simulink library "VehDynaPlayGround"  (R2024b)
settings: Solver=VariableStepAuto  StartTime=0.0  StopTime=10.0  RelTol=1e-3
undefined symbols (not defined in the file or in its folder): A_F, C_af, C_ar, C_d, f, g, h_aero, h_gc, InitialX, InitialY, Iz, lf, lr, m, Nf, Nr, phi, r_stat, r_w, rho, theta, V_wind
libraries: slpidlib x5
(part 1 of 3)
settings Model: Creator=headl  LastModifiedBy=headl

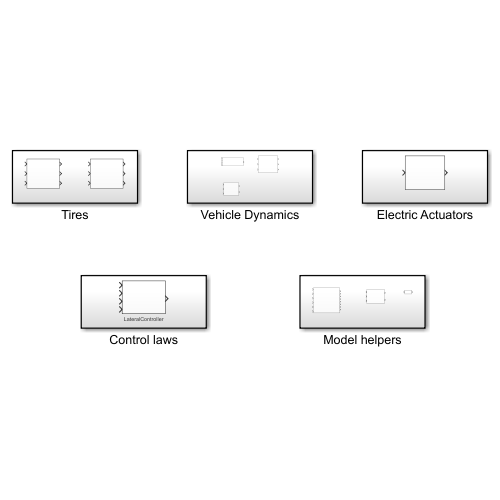
[thumbnail: Simulink's stored preview of the top-level diagram]
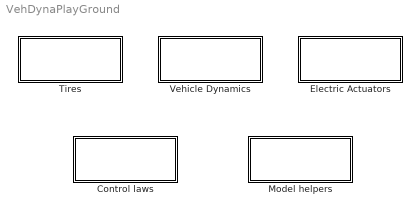
== system VehDynaPlayGround ==
  Control laws : Subsystem
  Electric Actuators : Subsystem
  Model helpers : Subsystem
  Tires : Subsystem
  Vehicle Dynamics : Subsystem

== system VehDynaPlayGround/Control laws ==
  LateralController : Subsystem  Variant=on  VariantControlMode=label  LabelModeActiveChoice=PID controller
      mask Display: image('$imagefile'); % Use "Edit Image" on toolstrip to change.

== system VehDynaPlayGround/Electric Actuators ==
  SteeringActuator : Subsystem  Variant=on  VariantControlMode=label  LabelModeActiveChoice=BLDC electric motor

== system VehDynaPlayGround/Model helpers ==
  CoordConvertRotation : Subsystem
      mask Display: image('$imagefile'); % Use "Edit Image" on toolstrip to change.
  GetRefference : MATLAB Function  TreatAsAtomicUnit=on  SystemSampleTime=0.05
  Wrap2pi : MATLAB Function  TreatAsAtomicUnit=on

== system VehDynaPlayGround/Tires ==
  Tyre ModelV1 : Subsystem
      mask Display: image('tire1_1.png');
  Tyre ModelV2 : Subsystem
      mask Display: image('$imagefile'); % Use "Edit Image" on toolstrip to change.

== system VehDynaPlayGround/Vehicle Dynamics ==
  LateralDynamics : Subsystem  Variant=on  VariantControlMode=label  LabelModeActiveChoice=Simplified Model
  LongitudinalDynamics : MATLAB Function  TreatAsAtomicUnit=on
  Transmission : MATLAB Function  TreatAsAtomicUnit=on

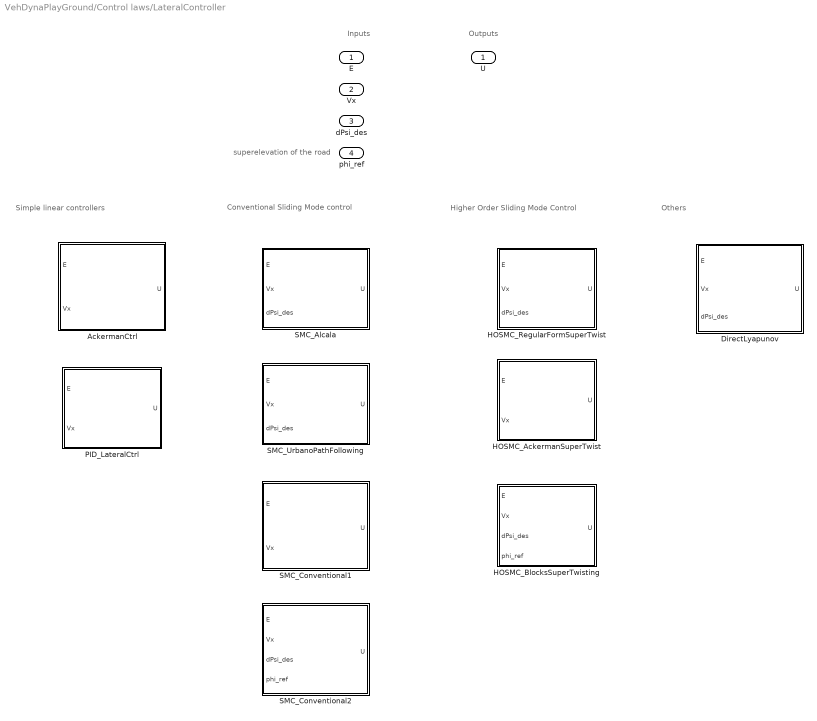
== system VehDynaPlayGround/Control laws/LateralController ==
  note: Others
  note: Higher Order Sliding Mode Control
  note: Conventional Sliding Mode control
  note: Simple linear controllers
  note: Outputs
  note: Inputs
  note: superelevation of the road
  E : Inport
  Vx : Inport  Port=2
  dPsi_des : Inport  Port=3
  phi_ref : Inport  Port=4
  AckermanCtrl : MATLAB Function  TreatAsAtomicUnit=on  VariantControl=Ackerman error feedback
  DirectLyapunov : MATLAB Function  TreatAsAtomicUnit=on  VariantControl=Direct Lyapunov Alcala et al.
  HOSMC_AckermanSuperTwist : Subsystem  VariantControl="HOSM  Ackerman + super twisting"
      mask Display: image('$imagefile'); % Use "Edit Image" on toolstrip to change.
  HOSMC_BlocksSuperTwisting : Subsystem  VariantControl=HOSM error feedback block +super twisting
      mask Display: image('$imagefile'); % Use "Edit Image" on toolstrip to change.
  HOSMC_RegularFormSuperTwist : Subsystem  VariantControl=HOSM regular form +super twisting
      mask Display: image('$imagefile'); % Use "Edit Image" on toolstrip to change.
  PID_LateralCtrl : Subsystem  VariantControl=PID controller
      mask Display: image('$imagefile'); % Use "Edit Image" on toolstrip to change.
  SMC_Alcala : Subsystem  VariantControl=Sliding mode Alcala et al.
      mask Display: image('$imagefile'); % Use "Edit Image" on toolstrip to change.
  SMC_Conventional1 : MATLAB Function  TreatAsAtomicUnit=on  VariantControl=SMC conventional V1
  SMC_Conventional2 : MATLAB Function  TreatAsAtomicUnit=on  VariantControl=SMC conventional V2
  SMC_UrbanoPathFollowing : Subsystem  VariantControl=Sliding mode Urbano path following
      mask Display: image('$imagefile'); % Use "Edit Image" on toolstrip to change.
  U : Outport

== system VehDynaPlayGround/Electric Actuators/SteeringActuator ==
  dd_ref : Inport
  BLDC_AngleCtrl : Subsystem  VariantControl=BLDC electric motor
      mask Display: image('$imagefile'); % Use "Edit Image" on toolstrip to change.
  NoActuator : Subsystem  VariantControl=No Actuator
  genericTransferFunction : Subsystem  VariantControl=Generic transfer function
      mask Display: image('$imagefile'); % Use "Edit Image" on toolstrip to change.
  dd_ctrl : Outport

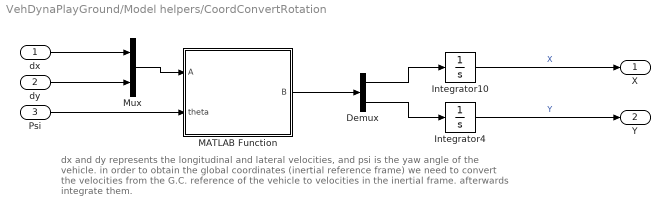
== system VehDynaPlayGround/Model helpers/CoordConvertRotation ==
  note: dx and dy represents the longitudinal and lateral velocities, and psi is the yaw angle of the vehicle. in order to obtain the global coordinates (inertial reference frame) we need to convert the velocities from the G.C. reference of the vehicle to velocities in the inertial frame. afterwards integrate them.
  dx : Inport
  dy : Inport  Port=2
  Psi : Inport  Port=3
  Demux : Demux  Outputs=2
  Integrator10 : Integrator  InitialCondition=InitialX
  Integrator4 : Integrator  InitialCondition=InitialY
  MATLAB Function : MATLAB Function  TreatAsAtomicUnit=on
  Mux : Mux  Inputs=2
  X : Outport  VectorParamsAs1DForOutWhenUnconnected=off
  Y : Outport  Port=2  VectorParamsAs1DForOutWhenUnconnected=off
  wires:
  Integrator10/1 -> X/1  "X"
  Integrator4/1 -> Y/1  "Y"
  Psi/1 -> MATLAB Function/2(theta)
  dx/1 -> Mux/1
  dy/1 -> Mux/2
  Mux/1 -> MATLAB Function/1(A)
  MATLAB Function/1(B) -> Demux/1
  Demux/1 -> Integrator10/1
  Demux/2 -> Integrator4/1

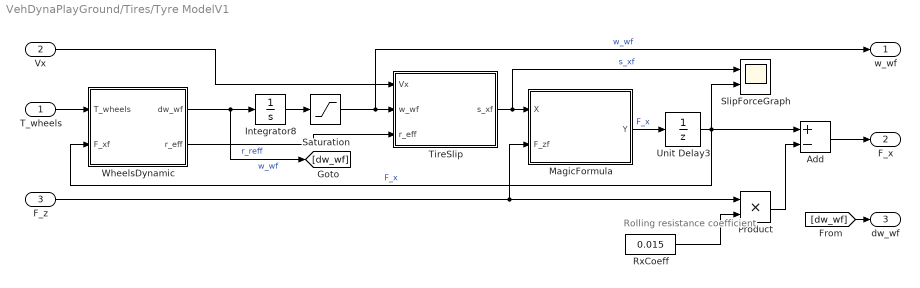
== system VehDynaPlayGround/Tires/Tyre ModelV1 ==
  note: Rolling resistance
      | coefficient
  T_wheels : Inport
  Vx : Inport  Port=2
  F_z : Inport  Port=3
  Add : Sum  Inputs=+-
  Integrator8 : Integrator
  MagicFormula : MATLAB Function  TreatAsAtomicUnit=on
  Product : Product
  RxCoeff : Constant  Value=0.015
  Saturation : Saturate  UpperLimit=100000  LowerLimit=0
  SlipForceGraph : Scope  NumInputPorts=2
  TireSlip : MATLAB Function  TreatAsAtomicUnit=on
  Unit Delay3 : UnitDelay  SampleTime=-1  HasFrameUpgradeWarning=on
  WheelsDynamic : MATLAB Function  TreatAsAtomicUnit=on
  w_wf : Outport
  F_x : Outport  Port=2
  dw_wf : Outport  Port=3
  wires:
  T_wheels/1 -> WheelsDynamic/1(T_wheels)
  Saturation/1 -> w_wf/1, TireSlip/2(w_wf)  "w_wf"
  WheelsDynamic/2(r_eff) -> TireSlip/3(r_eff)  "r_reff"
  MagicFormula/1(Y) -> Unit Delay3/1  "F_x"
  TireSlip/1(s_xf) -> SlipForceGraph/1, MagicFormula/1(X)  "s_xf"
  Integrator8/1 -> Saturation/1
  Vx/1 -> TireSlip/1(Vx)
  [dw_wf] -> dw_wf/1
  WheelsDynamic/1(dw_wf) -> [dw_wf], Integrator8/1  "w_wf"
  Add/1 -> F_x/1
  Product/1 -> Add/2
  F_z/1 -> Product/1, MagicFormula/2(F_zf)
  Unit Delay3/1 -> Add/1, SlipForceGraph/2, WheelsDynamic/2(F_xf)  "F_x"
  RxCoeff/1 -> Product/2

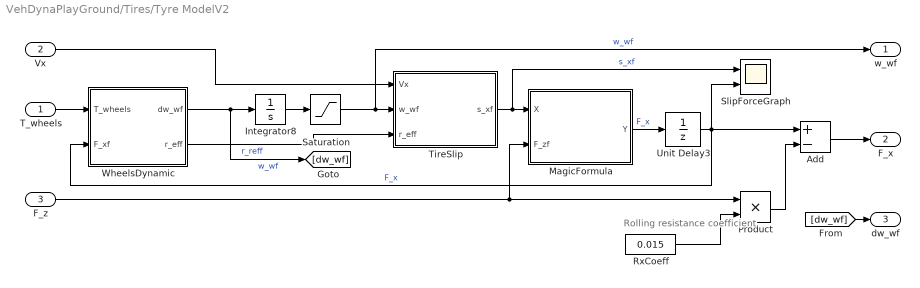
== system VehDynaPlayGround/Tires/Tyre ModelV2 ==
  note: Rolling resistance
      | coefficient
  T_wheels : Inport
  Vx : Inport  Port=2
  F_z : Inport  Port=3
  Add : Sum  Inputs=+-
  Integrator8 : Integrator
  MagicFormula : MATLAB Function  TreatAsAtomicUnit=on
  Product : Product
  RxCoeff : Constant  Value=0.015
  Saturation : Saturate  UpperLimit=100000  LowerLimit=0
  SlipForceGraph : Scope  NumInputPorts=2
  TireSlip : MATLAB Function  TreatAsAtomicUnit=on
  Unit Delay3 : UnitDelay  SampleTime=-1  HasFrameUpgradeWarning=on
  WheelsDynamic : MATLAB Function  TreatAsAtomicUnit=on
  w_wf : Outport
  F_x : Outport  Port=2
  dw_wf : Outport  Port=3
  wires:
  T_wheels/1 -> WheelsDynamic/1(T_wheels)
  Saturation/1 -> w_wf/1, TireSlip/2(w_wf)  "w_wf"
  WheelsDynamic/2(r_eff) -> TireSlip/3(r_eff)  "r_reff"
  MagicFormula/1(Y) -> Unit Delay3/1  "F_x"
  TireSlip/1(s_xf) -> SlipForceGraph/1, MagicFormula/1(X)  "s_xf"
  Integrator8/1 -> Saturation/1
  Vx/1 -> TireSlip/1(Vx)
  [dw_wf] -> dw_wf/1
  WheelsDynamic/1(dw_wf) -> [dw_wf], Integrator8/1  "w_wf"
  Add/1 -> F_x/1
  Product/1 -> Add/2
  F_z/1 -> Product/1, MagicFormula/2(F_zf)
  Unit Delay3/1 -> Add/1, SlipForceGraph/2, WheelsDynamic/2(F_xf)  "F_x"
  RxCoeff/1 -> Product/2

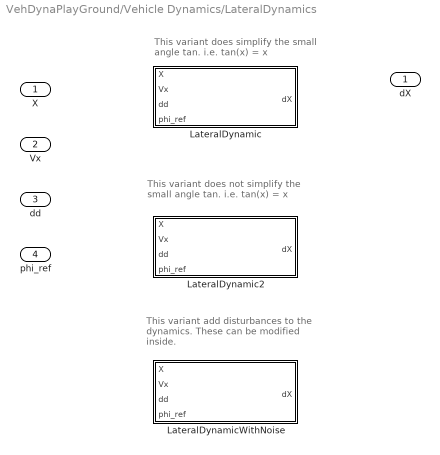
== system VehDynaPlayGround/Vehicle Dynamics/LateralDynamics ==
  note: This variant does not simplify the small angle tan. i.e. tan(x) = x
  note: This variant does simplify the small angle tan. i.e. tan(x) = x
  note: This variant add disturbances to the dynamics. These can be modified inside.
  X : Inport
  Vx : Inport  Port=2
  dd : Inport  Port=3
  phi_ref : Inport  Port=4
  LateralDynamic : MATLAB Function  TreatAsAtomicUnit=on  VariantControl=Simplified Model
  LateralDynamic2 : MATLAB Function  TreatAsAtomicUnit=on  VariantControl=Not Simplified Model
  LateralDynamicWithNoise : Subsystem  VariantControl=Lateral dynamic with disturbances
      mask Display: image('$imagefile'); % Use "Edit Image" on toolstrip to change.
  dX : Outport

== system VehDynaPlayGround/Control laws/LateralController/HOSMC_AckermanSuperTwist ==
  E : Inport
  Vx : Inport  Port=2
  HOSMC_AckermanSuperTwis1 : MATLAB Function  TreatAsAtomicUnit=on  VariantControl=SMC conventional
  Integrator1 : Integrator
  U : Outport
  wires:
  HOSMC_AckermanSuperTwis1/1(U) -> U/1
  E/1 -> HOSMC_AckermanSuperTwis1/1(E)
  Vx/1 -> HOSMC_AckermanSuperTwis1/2(Vx)
  HOSMC_AckermanSuperTwis1/2(dMu1) -> Integrator1/1
  Integrator1/1 -> HOSMC_AckermanSuperTwis1/3(Mu1)

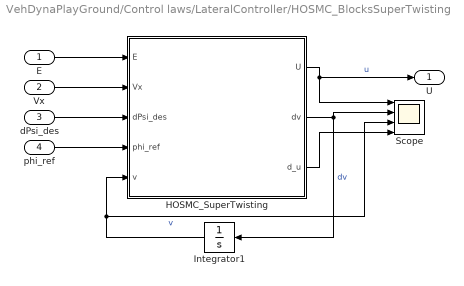
== system VehDynaPlayGround/Control laws/LateralController/HOSMC_BlocksSuperTwisting ==
  E : Inport
  Vx : Inport  Port=2
  dPsi_des : Inport  Port=3
  phi_ref : Inport  Port=4
  HOSMC_SuperTwisting : MATLAB Function  TreatAsAtomicUnit=on  VariantControl=SMC conventional
  Integrator1 : Integrator
  Scope : Scope  NumInputPorts=4
  U : Outport
  wires:
  HOSMC_SuperTwisting/1(U) -> U/1, Scope/1  "u"
  E/1 -> HOSMC_SuperTwisting/1(E)
  Vx/1 -> HOSMC_SuperTwisting/2(Vx)
  HOSMC_SuperTwisting/2(dv) -> Integrator1/1, Scope/2  "dv"
  Integrator1/1 -> Scope/3, HOSMC_SuperTwisting/5(v)  "v"
  dPsi_des/1 -> HOSMC_SuperTwisting/3(dPsi_des)
  phi_ref/1 -> HOSMC_SuperTwisting/4(phi_ref)
  HOSMC_SuperTwisting/3(d_u) -> Scope/4

== system VehDynaPlayGround/Control laws/LateralController/HOSMC_RegularFormSuperTwist ==
  E : Inport
  Vx : Inport  Port=2
  dPsi_des : Inport  Port=3
  HOSMC_RegularFormSuperTwist : MATLAB Function  TreatAsAtomicUnit=on  VariantControl=SMC conventional
  Integrator1 : Integrator
  Scope : Scope  NumInputPorts=3
  U : Outport
  wires:
  HOSMC_RegularFormSuperTwist/1(U) -> Scope/1, U/1
  E/1 -> HOSMC_RegularFormSuperTwist/1(E)
  Vx/1 -> HOSMC_RegularFormSuperTwist/2(Vx)
  HOSMC_RegularFormSuperTwist/2(dMu1) -> Integrator1/1, Scope/2
  Integrator1/1 -> Scope/3, HOSMC_RegularFormSuperTwist/4(Mu1)
  dPsi_des/1 -> HOSMC_RegularFormSuperTwist/3(dPsi_des)

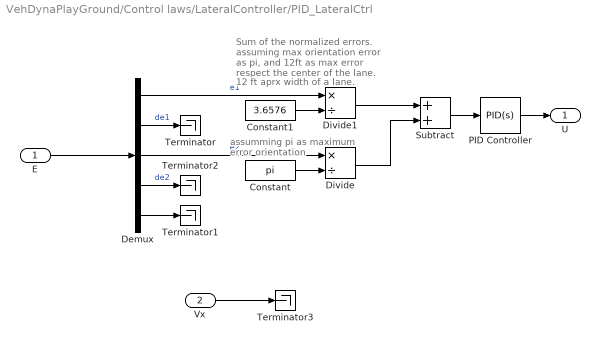
== system VehDynaPlayGround/Control laws/LateralController/PID_LateralCtrl ==
  note: Sum of the normalized errors. assuming max orientation error as pi, and 12ft as max error respect the center of the lane.
  note: assumming pi as maximum error orientation
  note: 12 ft aprx width of a lane.
  E : Inport
  Vx : Inport  Port=2
  Constant : Constant  Value=pi
  Constant1 : Constant  Value=3.6576
  Demux : Demux  Outputs=5
  Divide : Product  Inputs=*/
  Divide1 : Product  Inputs=*/
  PID Controller : slpidlib/PID Controller  Controller=PID  Form=Parallel  TimeDomain=Continuous-time  UseExternalTs=off  SampleTime=-1  IntegratorMethod=Forward Euler  FilterMethod=Forward Euler  ControllerParametersSource=internal  P=-10.4366715621745  I=-1.38825323496777  UseKiTs=off  D=1.48027109324461  UseExternalDerivativeSource=off  N=1.62687524156854  UseFilter=on  TunerSelectOption=Transfer Function Based (PID Tuner App)  InitialConditionSource=internal  InitialConditionForIntegrator=0  InitialConditionForFilter=0  DifferentiatorICPrevScaledInput=0  ExternalReset=none  TrackingMode=off  Kt=1  LimitOutput=off  SatLimitsSource=internal  UpperSaturationLimit=inf  LowerSaturationLimit=-inf  LinearizeAsGain=on  AntiWindupMode=none  Kb=1  LimitIntegrator=off  UpperIntegratorSaturationLimit=inf  LowerIntegratorSaturationLimit=-inf  POutMin=[]  POutMax=[]  IOutMin=[]  IOutMax=[]  DOutMin=[]  DOutMax=[]  NOutMin=[]  NOutMax=[]  SumOutMin=[]  SumOutMax=[]  SaturationOutMin=[]  SaturationOutMax=[]  PParamMin=[]  PParamMax=[]  IParamMin=[]  IParamMax=[]  DParamMin=[]  DParamMax=[]  NParamMin=[]  NParamMax=[]  KbParamMin=[]  KbParamMax=[]  KtParamMin=[]  KtParamMax=[]  KbOutMin=[]  KbOutMax=[]  KtOutMin=[]  KtOutMax=[]  IntegratorOutMin=[]  IntegratorOutMax=[]  FilterOutMin=[]  FilterOutMax=[]  SumI1OutMin=[]  SumI1OutMax=[]  SumI2OutMin=[]  SumI2OutMax=[]  SumI3OutMin=[]  SumI3OutMax=[]  SumI4OutMin=[]  SumI4OutMax=[]  SumDOutMin=[]  SumDOutMax=[]  DifferentiatorOutMin=[]  DifferentiatorOutMax=[]  FilterDiffOutCoefMin=[]  FilterDiffOutCoefMax=[]  ReciprocalOutMin=[]  ReciprocalOutMax=[]  SumDenOutMin=[]  SumDenOutMax=[]  SumNumOutMin=[]  SumNumOutMax=[]  DivideOutMin=[]  DivideOutMax=[]  UdiffTsProdOutMin=[]  UdiffTsProdOutMax=[]  NTsProdOutMin=[]  NTsProdOutMax=[]  UintegralTsProdOutMin=[]  UintegralTsProdOutMax=[]  UngainTsProdOutMin=[]  UngainTsProdOutMax=[]  ClampingZeroOutDataTypeStr=Inherit: Inherit via back propagation  ClampingZeroOutMin=[]  ClampingZeroOutMax=[]  FilterDenConstantOutDataTypeStr=Inherit: Inherit via back propagation  FilterDenConstantOutMin=[]  FilterDenConstantOutMax=[]  PCopyOutDataTypeStr=Inherit: Inherit via back propagation  PCopyOutMin=[]  PCopyOutMax=[]  NCopyOutDataTypeStr=Inherit: Inherit via back propagation  NCopyOutMin=[]  NCopyOutMax=[]  IntegratorContinuousStateAttributes=''  IntegratorStateMustResolveToSignalObject=off  IntegratorRTWStateStorageClass=Auto  FilterContinuousStateAttributes=''  FilterStateMustResolveToSignalObject=off  FilterRTWStateStorageClass=Auto  ParallelPVariant=InternalParameters  IdealPVariant=Disabled  IVariant=InternalParameters  DVariant=InternalParameters  IntegratorVariant=Continuous  SatVariant=Disabled  AWVariant=Passthrough  PCopyVariant=Disabled  TRVariant=Disabled  FdbkBlocksVariant=Forward  IdealPFdbkVariant=Disabled  SatFdbkVariant=Disabled  DerivativeFilterVariant=ContFilter  NVariant=InternalParameters  NCopyVariant=Disabled  FilterICVariant=InternalICsFilter  IntegratorICVariant=InternalICs  ExternalResetVariant=Disabled  TRSumVariant=Passthrough  SumFdbkVariant=Disabled  SumVariant=Sum_PID  TsampFilterVariant=InternalTs  TsampNgainVariant=Passthrough  TsampIntegralVariant=Disabled_SignalSpec  ExternalSaturationOutDataTypeStr=Inherit: Same as second input  DerivativeSourceVariant=ErrorSignal  PreIntVariant=InternalPreInt
  Subtract : Sum
  Terminator{,1..3} (4 alike) : Terminator
  U : Outport
  wires:
  E/1 -> Demux/1
  Demux/2 -> Terminator/1  "de1"
  Demux/4 -> Terminator2/1  "de2"
  Vx/1 -> Terminator3/1
  Subtract/1 -> PID Controller/1
  PID Controller/1 -> U/1
  Demux/3 -> Divide/1  "e2"
  Divide/1 -> Subtract/2
  Constant/1 -> Divide/2
  Demux/1 -> Divide1/1  "e1"
  Constant1/1 -> Divide1/2
  Divide1/1 -> Subtract/1
  Demux/5 -> Terminator1/1

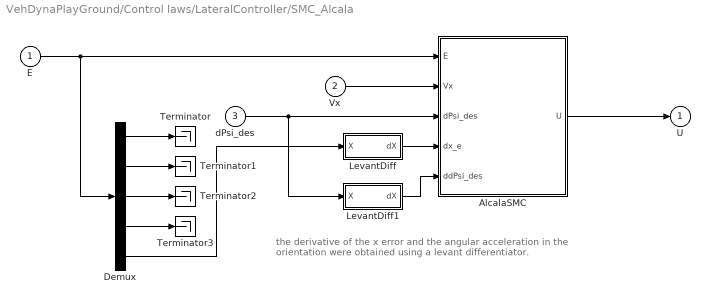
== system VehDynaPlayGround/Control laws/LateralController/SMC_Alcala ==
  note: the derivative of the x error and the angular acceleration in the orientation were obtained using a levant differentiator.
  E : Inport
  Vx : Inport  Port=2
  dPsi_des : Inport  Port=3
  AlcalaSMC : MATLAB Function  TreatAsAtomicUnit=on  VariantControl=Sliding mode Ctrl 1
  Demux : Demux  Outputs=5
  LevantDiff : Subsystem  mask{lambda1=60, alpha1=2000}
      mask prompts: lambda1 "Lambda :"; alpha1 "Alpha    :"
      mask help: Levant differenciator
      mask Help: This is based on Levant A. (1998). Robust exact differentiation via sliding mode technique. Automatica, 34(3), 379-384
  LevantDiff1 : Subsystem  mask{lambda1=60, alpha1=2000}
      mask prompts: lambda1 "Lambda :"; alpha1 "Alpha    :"
      mask help: Levant differenciator
      mask Help: This is based on Levant A. (1998). Robust exact differentiation via sliding mode technique. Automatica, 34(3), 379-384
  Terminator{,1..3} (4 alike) : Terminator
  U : Outport
  wires:
  E/1 -> Demux/1, AlcalaSMC/1(E)
  Vx/1 -> AlcalaSMC/2(Vx)
  dPsi_des/1 -> LevantDiff1/1(X), AlcalaSMC/3(dPsi_des)
  AlcalaSMC/1(U) -> U/1
  Demux/1 -> Terminator/1
  Demux/2 -> Terminator1/1
  Demux/3 -> Terminator2/1
  Demux/4 -> Terminator3/1
  LevantDiff/1(dX) -> AlcalaSMC/4(dx_e)
  Demux/5 -> LevantDiff/1(X)
  LevantDiff1/1(dX) -> AlcalaSMC/5(ddPsi_des)

== system VehDynaPlayGround/Control laws/LateralController/SMC_UrbanoPathFollowing ==
  E : Inport
  Vx : Inport  Port=2
  dPsi_des : Inport  Port=3
  Integrator : Integrator
  SMC_UrbanoPathFollowing : MATLAB Function  TreatAsAtomicUnit=on  VariantControl=Sliding mode Urbano Path Following
  U : Outport
  wires:
  SMC_UrbanoPathFollowing/1(U) -> U/1
  E/1 -> SMC_UrbanoPathFollowing/1(E)
  Vx/1 -> SMC_UrbanoPathFollowing/2(Vx)
  dPsi_des/1 -> SMC_UrbanoPathFollowing/3(dPsi_des)
  SMC_UrbanoPathFollowing/2(dd_d) -> Integrator/1
  Integrator/1 -> SMC_UrbanoPathFollowing/4(d_d)

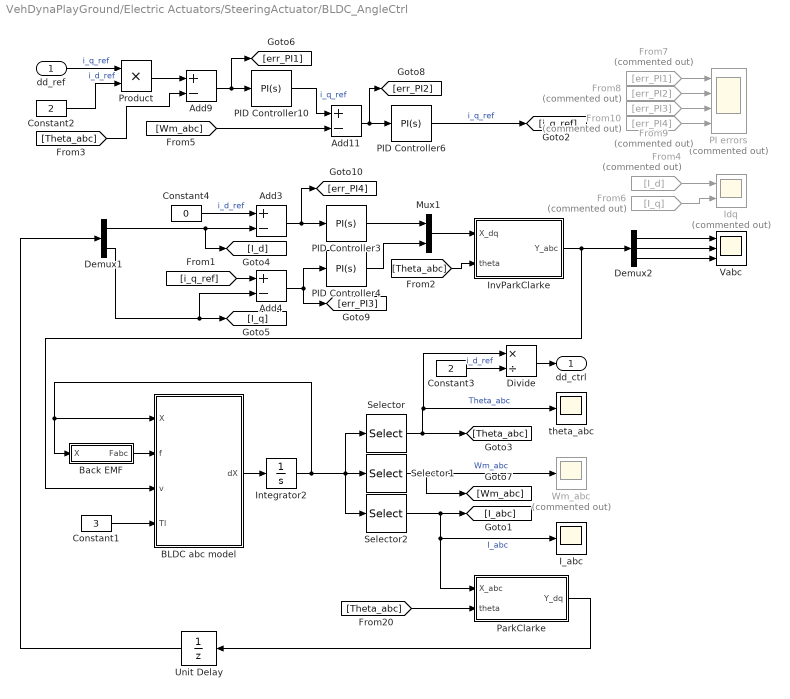
== system VehDynaPlayGround/Electric Actuators/SteeringActuator/BLDC_AngleCtrl ==
  dd_ref : Inport
  Add{3..4,9,11} (4 alike) : Sum  Inputs=+-
  BLDC abc model : MATLAB Function  TreatAsAtomicUnit=on
  Back EMF : MATLAB Function  TreatAsAtomicUnit=on
  Constant1 : Constant  Value=3
  Constant2 : Constant  Value=2
  Constant3 : Constant  Value=2
  Constant4 : Constant  Value=0
  Demux1 : Demux  Outputs=2
  Demux2 : Demux  Outputs=3
  Divide : Product  Inputs=*/
  From10 : From  Commented=on  GotoTag=err_PI4
  From4 : From  Commented=on  GotoTag=I_d
  From6 : From  Commented=on  GotoTag=I_q
  From7 : From  Commented=on  GotoTag=err_PI1
  From8 : From  Commented=on  GotoTag=err_PI2
  From9 : From  Commented=on  GotoTag=err_PI3
  I_abc : Scope
  Idq : Scope  Commented=on  NumInputPorts=2
  Integrator2 : Integrator  InitialCondition=[0;0;0;0.1;0]
  InvParkClarke : MATLAB Function  TreatAsAtomicUnit=on
  Mux1 : Mux  Inputs=2
  PI errors : Scope  Commented=on  NumInputPorts=4
  PID Controller10 : slpidlib/PID Controller  Controller=PI  Form=Parallel  TimeDomain=Continuous-time  UseExternalTs=off  SampleTime=-1  IntegratorMethod=Forward Euler  FilterMethod=Forward Euler  ControllerParametersSource=internal  P=21.2472922845302  I=1497.59558537531  UseKiTs=off  D=0  UseExternalDerivativeSource=off  N=100  UseFilter=on  TunerSelectOption=Transfer Function Based (PID Tuner App)  InitialConditionSource=internal  InitialConditionForIntegrator=0  InitialConditionForFilter=0  DifferentiatorICPrevScaledInput=0  ExternalReset=none  TrackingMode=off  Kt=1  LimitOutput=off  SatLimitsSource=internal  UpperSaturationLimit=inf  LowerSaturationLimit=-inf  LinearizeAsGain=on  AntiWindupMode=none  Kb=1  LimitIntegrator=off  UpperIntegratorSaturationLimit=inf  LowerIntegratorSaturationLimit=-inf  POutMin=[]  POutMax=[]  IOutMin=[]  IOutMax=[]  DOutMin=[]  DOutMax=[]  NOutMin=[]  NOutMax=[]  SumOutMin=[]  SumOutMax=[]  SaturationOutMin=[]  SaturationOutMax=[]  PParamMin=[]  PParamMax=[]  IParamMin=[]  IParamMax=[]  DParamMin=[]  DParamMax=[]  NParamMin=[]  NParamMax=[]  KbParamMin=[]  KbParamMax=[]  KtParamMin=[]  KtParamMax=[]  KbOutMin=[]  KbOutMax=[]  KtOutMin=[]  KtOutMax=[]  IntegratorOutMin=[]  IntegratorOutMax=[]  FilterOutMin=[]  FilterOutMax=[]  SumI1OutMin=[]  SumI1OutMax=[]  SumI2OutMin=[]  SumI2OutMax=[]  SumI3OutMin=[]  SumI3OutMax=[]  SumI4OutMin=[]  SumI4OutMax=[]  SumDOutMin=[]  SumDOutMax=[]  DifferentiatorOutMin=[]  DifferentiatorOutMax=[]  FilterDiffOutCoefMin=[]  FilterDiffOutCoefMax=[]  ReciprocalOutMin=[]  ReciprocalOutMax=[]  SumDenOutMin=[]  SumDenOutMax=[]  SumNumOutMin=[]  SumNumOutMax=[]  DivideOutMin=[]  DivideOutMax=[]  UdiffTsProdOutMin=[]  UdiffTsProdOutMax=[]  NTsProdOutMin=[]  NTsProdOutMax=[]  UintegralTsProdOutMin=[]  UintegralTsProdOutMax=[]  UngainTsProdOutMin=[]  UngainTsProdOutMax=[]  ClampingZeroOutDataTypeStr=Inherit: Inherit via back propagation  ClampingZeroOutMin=[]  ClampingZeroOutMax=[]  FilterDenConstantOutDataTypeStr=Inherit: Inherit via back propagation  FilterDenConstantOutMin=[]  FilterDenConstantOutMax=[]  PCopyOutDataTypeStr=Inherit: Inherit via back propagation  PCopyOutMin=[]  PCopyOutMax=[]  NCopyOutDataTypeStr=Inherit: Inherit via back propagation  NCopyOutMin=[]  NCopyOutMax=[]  IntegratorContinuousStateAttributes=''  IntegratorStateMustResolveToSignalObject=off  IntegratorRTWStateStorageClass=Auto  FilterContinuousStateAttributes=''  FilterStateMustResolveToSignalObject=off  FilterRTWStateStorageClass=Auto  ParallelPVariant=InternalParameters  IdealPVariant=Disabled  IVariant=InternalParameters  DVariant=Disabled  IntegratorVariant=Continuous  SatVariant=Disabled  AWVariant=Passthrough  PCopyVariant=Disabled  TRVariant=Disabled  FdbkBlocksVariant=Forward  IdealPFdbkVariant=Disabled  SatFdbkVariant=Disabled  DerivativeFilterVariant=Disabled  NVariant=Disabled  NCopyVariant=Disabled_SignalSpec  FilterICVariant=Disabled  IntegratorICVariant=InternalICs  ExternalResetVariant=Disabled  TRSumVariant=Passthrough  SumFdbkVariant=Disabled  SumVariant=Sum_PI  TsampFilterVariant=InternalTs  TsampNgainVariant=Passthrough  TsampIntegralVariant=Disabled_SignalSpec  ExternalSaturationOutDataTypeStr=Inherit: Same as second input  DerivativeSourceVariant=Disabled  PreIntVariant=InternalPreInt
  PID Controller3 : slpidlib/PID Controller  Controller=PI  Form=Parallel  TimeDomain=Continuous-time  UseExternalTs=off  SampleTime=-1  IntegratorMethod=Forward Euler  FilterMethod=Forward Euler  ControllerParametersSource=internal  P=70  I=0.3  UseKiTs=off  D=0  UseExternalDerivativeSource=off  N=100  UseFilter=on  TunerSelectOption=Transfer Function Based (PID Tuner App)  InitialConditionSource=internal  InitialConditionForIntegrator=0  InitialConditionForFilter=0  DifferentiatorICPrevScaledInput=0  ExternalReset=none  TrackingMode=off  Kt=1  LimitOutput=off  SatLimitsSource=internal  UpperSaturationLimit=inf  LowerSaturationLimit=-inf  LinearizeAsGain=on  AntiWindupMode=none  Kb=1  LimitIntegrator=off  UpperIntegratorSaturationLimit=inf  LowerIntegratorSaturationLimit=-inf  POutMin=[]  POutMax=[]  IOutMin=[]  IOutMax=[]  DOutMin=[]  DOutMax=[]  NOutMin=[]  NOutMax=[]  SumOutMin=[]  SumOutMax=[]  SaturationOutMin=[]  SaturationOutMax=[]  PParamMin=[]  PParamMax=[]  IParamMin=[]  IParamMax=[]  DParamMin=[]  DParamMax=[]  NParamMin=[]  NParamMax=[]  KbParamMin=[]  KbParamMax=[]  KtParamMin=[]  KtParamMax=[]  KbOutMin=[]  KbOutMax=[]  KtOutMin=[]  KtOutMax=[]  IntegratorOutMin=[]  IntegratorOutMax=[]  FilterOutMin=[]  FilterOutMax=[]  SumI1OutMin=[]  SumI1OutMax=[]  SumI2OutMin=[]  SumI2OutMax=[]  SumI3OutMin=[]  SumI3OutMax=[]  SumI4OutMin=[]  SumI4OutMax=[]  SumDOutMin=[]  SumDOutMax=[]  DifferentiatorOutMin=[]  DifferentiatorOutMax=[]  FilterDiffOutCoefMin=[]  FilterDiffOutCoefMax=[]  ReciprocalOutMin=[]  ReciprocalOutMax=[]  SumDenOutMin=[]  SumDenOutMax=[]  SumNumOutMin=[]  SumNumOutMax=[]  DivideOutMin=[]  DivideOutMax=[]  UdiffTsProdOutMin=[]  UdiffTsProdOutMax=[]  NTsProdOutMin=[]  NTsProdOutMax=[]  UintegralTsProdOutMin=[]  UintegralTsProdOutMax=[]  UngainTsProdOutMin=[]  UngainTsProdOutMax=[]  ClampingZeroOutDataTypeStr=Inherit: Inherit via back propagation  ClampingZeroOutMin=[]  ClampingZeroOutMax=[]  FilterDenConstantOutDataTypeStr=Inherit: Inherit via back propagation  FilterDenConstantOutMin=[]  FilterDenConstantOutMax=[]  PCopyOutDataTypeStr=Inherit: Inherit via back propagation  PCopyOutMin=[]  PCopyOutMax=[]  NCopyOutDataTypeStr=Inherit: Inherit via back propagation  NCopyOutMin=[]  NCopyOutMax=[]  IntegratorContinuousStateAttributes=''  IntegratorStateMustResolveToSignalObject=off  IntegratorRTWStateStorageClass=Auto  FilterContinuousStateAttributes=''  FilterStateMustResolveToSignalObject=off  FilterRTWStateStorageClass=Auto  ParallelPVariant=InternalParameters  IdealPVariant=Disabled  IVariant=InternalParameters  DVariant=Disabled  IntegratorVariant=Continuous  SatVariant=Disabled  AWVariant=Passthrough  PCopyVariant=Disabled  TRVariant=Disabled  FdbkBlocksVariant=Forward  IdealPFdbkVariant=Disabled  SatFdbkVariant=Disabled  DerivativeFilterVariant=Disabled  NVariant=Disabled  NCopyVariant=Disabled_SignalSpec  FilterICVariant=Disabled  IntegratorICVariant=InternalICs  ExternalResetVariant=Disabled  TRSumVariant=Passthrough  SumFdbkVariant=Disabled  SumVariant=Sum_PI  TsampFilterVariant=InternalTs  TsampNgainVariant=Passthrough  TsampIntegralVariant=Disabled_SignalSpec  ExternalSaturationOutDataTypeStr=Inherit: Same as second input  DerivativeSourceVariant=Disabled  PreIntVariant=InternalPreInt
  PID Controller4 : slpidlib/PID Controller  Controller=PI  Form=Parallel  TimeDomain=Continuous-time  UseExternalTs=off  SampleTime=-1  IntegratorMethod=Forward Euler  FilterMethod=Forward Euler  ControllerParametersSource=internal  P=70  I=0.3  UseKiTs=off  D=0  UseExternalDerivativeSource=off  N=100  UseFilter=on  TunerSelectOption=Transfer Function Based (PID Tuner App)  InitialConditionSource=internal  InitialConditionForIntegrator=0  InitialConditionForFilter=0  DifferentiatorICPrevScaledInput=0  ExternalReset=none  TrackingMode=off  Kt=1  LimitOutput=off  SatLimitsSource=internal  UpperSaturationLimit=inf  LowerSaturationLimit=-inf  LinearizeAsGain=on  AntiWindupMode=none  Kb=1  LimitIntegrator=off  UpperIntegratorSaturationLimit=inf  LowerIntegratorSaturationLimit=-inf  POutMin=[]  POutMax=[]  IOutMin=[]  IOutMax=[]  DOutMin=[]  DOutMax=[]  NOutMin=[]  NOutMax=[]  SumOutMin=[]  SumOutMax=[]  SaturationOutMin=[]  SaturationOutMax=[]  PParamMin=[]  PParamMax=[]  IParamMin=[]  IParamMax=[]  DParamMin=[]  DParamMax=[]  NParamMin=[]  NParamMax=[]  KbParamMin=[]  KbParamMax=[]  KtParamMin=[]  KtParamMax=[]  KbOutMin=[]  KbOutMax=[]  KtOutMin=[]  KtOutMax=[]  IntegratorOutMin=[]  IntegratorOutMax=[]  FilterOutMin=[]  FilterOutMax=[]  SumI1OutMin=[]  SumI1OutMax=[]  SumI2OutMin=[]  SumI2OutMax=[]  SumI3OutMin=[]  SumI3OutMax=[]  SumI4OutMin=[]  SumI4OutMax=[]  SumDOutMin=[]  SumDOutMax=[]  DifferentiatorOutMin=[]  DifferentiatorOutMax=[]  FilterDiffOutCoefMin=[]  FilterDiffOutCoefMax=[]  ReciprocalOutMin=[]  ReciprocalOutMax=[]  SumDenOutMin=[]  SumDenOutMax=[]  SumNumOutMin=[]  SumNumOutMax=[]  DivideOutMin=[]  DivideOutMax=[]  UdiffTsProdOutMin=[]  UdiffTsProdOutMax=[]  NTsProdOutMin=[]  NTsProdOutMax=[]  UintegralTsProdOutMin=[]  UintegralTsProdOutMax=[]  UngainTsProdOutMin=[]  UngainTsProdOutMax=[]  ClampingZeroOutDataTypeStr=Inherit: Inherit via back propagation  ClampingZeroOutMin=[]  ClampingZeroOutMax=[]  FilterDenConstantOutDataTypeStr=Inherit: Inherit via back propagation  FilterDenConstantOutMin=[]  FilterDenConstantOutMax=[]  PCopyOutDataTypeStr=Inherit: Inherit via back propagation  PCopyOutMin=[]  PCopyOutMax=[]  NCopyOutDataTypeStr=Inherit: Inherit via back propagation  NCopyOutMin=[]  NCopyOutMax=[]  IntegratorContinuousStateAttributes=''  IntegratorStateMustResolveToSignalObject=off  IntegratorRTWStateStorageClass=Auto  FilterContinuousStateAttributes=''  FilterStateMustResolveToSignalObject=off  FilterRTWStateStorageClass=Auto  ParallelPVariant=InternalParameters  IdealPVariant=Disabled  IVariant=InternalParameters  DVariant=Disabled  IntegratorVariant=Continuous  SatVariant=Disabled  AWVariant=Passthrough  PCopyVariant=Disabled  TRVariant=Disabled  FdbkBlocksVariant=Forward  IdealPFdbkVariant=Disabled  SatFdbkVariant=Disabled  DerivativeFilterVariant=Disabled  NVariant=Disabled  NCopyVariant=Disabled_SignalSpec  FilterICVariant=Disabled  IntegratorICVariant=InternalICs  ExternalResetVariant=Disabled  TRSumVariant=Passthrough  SumFdbkVariant=Disabled  SumVariant=Sum_PI  TsampFilterVariant=InternalTs  TsampNgainVariant=Passthrough  TsampIntegralVariant=Disabled_SignalSpec  ExternalSaturationOutDataTypeStr=Inherit: Same as second input  DerivativeSourceVariant=Disabled  PreIntVariant=InternalPreInt
  PID Controller6 : slpidlib/PID Controller  Controller=PI  Form=Parallel  TimeDomain=Continuous-time  UseExternalTs=off  SampleTime=-1  IntegratorMethod=Forward Euler  FilterMethod=Forward Euler  ControllerParametersSource=internal  P=-0.39820378606854  I=-44.4991237925307  UseKiTs=off  D=0  UseExternalDerivativeSource=off  N=100  UseFilter=on  TunerSelectOption=Transfer Function Based (PID Tuner App)  InitialConditionSource=internal  InitialConditionForIntegrator=0  InitialConditionForFilter=0  DifferentiatorICPrevScaledInput=0  ExternalReset=none  TrackingMode=off  Kt=1  LimitOutput=off  SatLimitsSource=internal  UpperSaturationLimit=inf  LowerSaturationLimit=-inf  LinearizeAsGain=on  AntiWindupMode=none  Kb=1  LimitIntegrator=off  UpperIntegratorSaturationLimit=inf  LowerIntegratorSaturationLimit=-inf  POutMin=[]  POutMax=[]  IOutMin=[]  IOutMax=[]  DOutMin=[]  DOutMax=[]  NOutMin=[]  NOutMax=[]  SumOutMin=[]  SumOutMax=[]  SaturationOutMin=[]  SaturationOutMax=[]  PParamMin=[]  PParamMax=[]  IParamMin=[]  IParamMax=[]  DParamMin=[]  DParamMax=[]  NParamMin=[]  NParamMax=[]  KbParamMin=[]  KbParamMax=[]  KtParamMin=[]  KtParamMax=[]  KbOutMin=[]  KbOutMax=[]  KtOutMin=[]  KtOutMax=[]  IntegratorOutMin=[]  IntegratorOutMax=[]  FilterOutMin=[]  FilterOutMax=[]  SumI1OutMin=[]  SumI1OutMax=[]  SumI2OutMin=[]  SumI2OutMax=[]  SumI3OutMin=[]  SumI3OutMax=[]  SumI4OutMin=[]  SumI4OutMax=[]  SumDOutMin=[]  SumDOutMax=[]  DifferentiatorOutMin=[]  DifferentiatorOutMax=[]  FilterDiffOutCoefMin=[]  FilterDiffOutCoefMax=[]  ReciprocalOutMin=[]  ReciprocalOutMax=[]  SumDenOutMin=[]  SumDenOutMax=[]  SumNumOutMin=[]  SumNumOutMax=[]  DivideOutMin=[]  DivideOutMax=[]  UdiffTsProdOutMin=[]  UdiffTsProdOutMax=[]  NTsProdOutMin=[]  NTsProdOutMax=[]  UintegralTsProdOutMin=[]  UintegralTsProdOutMax=[]  UngainTsProdOutMin=[]  UngainTsProdOutMax=[]  ClampingZeroOutDataTypeStr=Inherit: Inherit via back propagation  ClampingZeroOutMin=[]  ClampingZeroOutMax=[]  FilterDenConstantOutDataTypeStr=Inherit: Inherit via back propagation  FilterDenConstantOutMin=[]  FilterDenConstantOutMax=[]  PCopyOutDataTypeStr=Inherit: Inherit via back propagation  PCopyOutMin=[]  PCopyOutMax=[]  NCopyOutDataTypeStr=Inherit: Inherit via back propagation  NCopyOutMin=[]  NCopyOutMax=[]  IntegratorContinuousStateAttributes=''  IntegratorStateMustResolveToSignalObject=off  IntegratorRTWStateStorageClass=Auto  FilterContinuousStateAttributes=''  FilterStateMustResolveToSignalObject=off  FilterRTWStateStorageClass=Auto  ParallelPVariant=InternalParameters  IdealPVariant=Disabled  IVariant=InternalParameters  DVariant=Disabled  IntegratorVariant=Continuous  SatVariant=Disabled  AWVariant=Passthrough  PCopyVariant=Disabled  TRVariant=Disabled  FdbkBlocksVariant=Forward  IdealPFdbkVariant=Disabled  SatFdbkVariant=Disabled  DerivativeFilterVariant=Disabled  NVariant=Disabled  NCopyVariant=Disabled_SignalSpec  FilterICVariant=Disabled  IntegratorICVariant=InternalICs  ExternalResetVariant=Disabled  TRSumVariant=Passthrough  SumFdbkVariant=Disabled  SumVariant=Sum_PI  TsampFilterVariant=InternalTs  TsampNgainVariant=Passthrough  TsampIntegralVariant=Disabled_SignalSpec  ExternalSaturationOutDataTypeStr=Inherit: Same as second input  DerivativeSourceVariant=Disabled  PreIntVariant=InternalPreInt
  ParkClarke : MATLAB Function  TreatAsAtomicUnit=on
  Product : Product
  Selector : Selector  InputPortWidth=5  IndexOptions=Index vector (dialog)  Indices=[5]  OutputSizes=1
  Selector1 : Selector  InputPortWidth=5  IndexOptions=Index vector (dialog)  Indices=[4]  OutputSizes=1
  Selector2 : Selector  InputPortWidth=5  IndexOptions=Index vector (dialog)  Indices=[1:3]  OutputSizes=1
  Unit Delay : UnitDelay  InitialCondition=[0;0]  SampleTime=-1  HasFrameUpgradeWarning=on
  Vabc : Scope  NumInputPorts=3
  Wm_abc : Scope  Commented=on
  theta_abc : Scope
  dd_ctrl : Outport
  wires:
  PID Controller10/1 -> Add11/1  "i_q_ref"
  Constant4/1 -> Add3/1  "i_d_ref"
  Back EMF/1(Fabc) -> BLDC abc model/2(f)
  Unit Delay/1 -> Demux1/1
  Add11/1 -> PID Controller6/1, [err_PI2]
  Add9/1 -> [err_PI1], PID Controller10/1
  Demux1/2 -> [I_q], Add4/2
  [Wm_abc] -> Add11/2
  [Theta_abc] -> Add9/2
  Selector2/1 -> ParkClarke/1(X_abc), I_abc/1, [I_abc]  "I_abc"
  Mux1/1 -> InvParkClarke/1(X_dq)
  [Theta_abc] -> ParkClarke/2(theta)
  [Theta_abc] -> InvParkClarke/2(theta)
  Selector/1 -> [Theta_abc], Divide/1, theta_abc/1  "Theta_abc"
  PID Controller3/1 -> Mux1/1
  ParkClarke/1(Y_dq) -> Unit Delay/1
  Constant1/1 -> BLDC abc model/4(Tl)
  InvParkClarke/1(Y_abc) -> BLDC abc model/3(v), Demux2/1
  PID Controller4/1 -> Mux1/2
  BLDC abc model/1(dX) -> Integrator2/1
  Selector1/1 -> [Wm_abc], Wm_abc/1  "Wm_abc"
  Add4/1 -> [err_PI3], PID Controller4/1
  Demux1/1 -> [I_d], Add3/2
  Add3/1 -> [err_PI4], PID Controller3/1
  Integrator2/1 -> Selector2/1, Selector/1, Selector1/1, BLDC abc model/1(X), Back EMF/1(X)
  PID Controller6/1 -> [i_q_ref]  "i_q_ref"
  [i_q_ref] -> Add4/1
  Product/1 -> Add9/1
  dd_ref/1 -> Product/1  "i_q_ref"
  Constant2/1 -> Product/2  "i_d_ref"
  Divide/1 -> dd_ctrl/1
  Constant3/1 -> Divide/2  "i_d_ref"
  From4/1 -> Idq/1
  From6/1 -> Idq/2
  From7/1 -> PI errors/1
  From8/1 -> PI errors/2
  From9/1 -> PI errors/3
  From10/1 -> PI errors/4
  Demux2/1 -> Vabc/1
  Demux2/2 -> Vabc/2
  Demux2/3 -> Vabc/3

== system VehDynaPlayGround/Electric Actuators/SteeringActuator/NoActuator ==
  dd_ref : Inport
  dd_ctrl : Outport
  wires:
  dd_ref/1 -> dd_ctrl/1

== system VehDynaPlayGround/Electric Actuators/SteeringActuator/genericTransferFunction ==
  dd_ref : Inport
  TF_AlcalaUrbano : TransferFcn  Commented=on  Numerator=[(2*pi*5)^2]  Denominator=[1 2*0.7*(2*pi*5) (2*pi*5)^2]
  TF_BLDCIdentification : TransferFcn  Numerator=1552  Denominator=[1 18.95 1543]
  dd_ctrl : Outport
  wires:
  dd_ref/1 -> TF_BLDCIdentification/1
  TF_BLDCIdentification/1 -> dd_ctrl/1

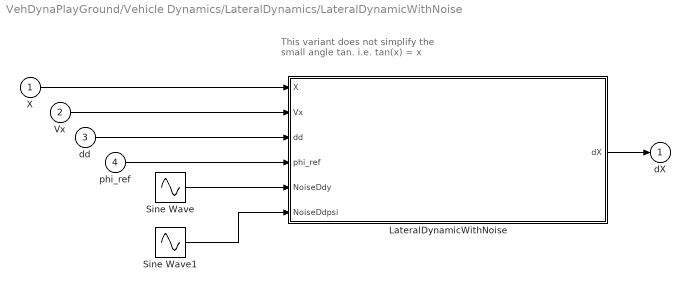
== system VehDynaPlayGround/Vehicle Dynamics/LateralDynamics/LateralDynamicWithNoise ==
  note: This variant does not simplify the small angle tan. i.e. tan(x) = x
  X : Inport
  Vx : Inport  Port=2
  dd : Inport  Port=3
  phi_ref : Inport  Port=4
  LateralDynamicWithNoise : MATLAB Function  TreatAsAtomicUnit=on  VariantControl=NotSimplifiedModel
  Sine Wave : Sin  Amplitude=0.6  Frequency=(2*pi)/8  SampleTime=0
  Sine Wave1 : Sin  Amplitude=pi/60  Frequency=pi/8  SampleTime=0
  dX : Outport
  wires:
  X/1 -> LateralDynamicWithNoise/1(X)
  Vx/1 -> LateralDynamicWithNoise/2(Vx)
  dd/1 -> LateralDynamicWithNoise/3(dd)
  LateralDynamicWithNoise/1(dX) -> dX/1
  phi_ref/1 -> LateralDynamicWithNoise/4(phi_ref)
  Sine Wave/1 -> LateralDynamicWithNoise/5(NoiseDdy)
  Sine Wave1/1 -> LateralDynamicWithNoise/6(NoiseDdpsi)

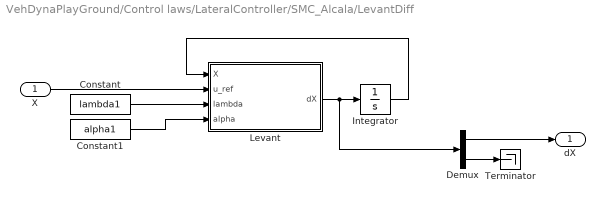
== system VehDynaPlayGround/Control laws/LateralController/SMC_Alcala/LevantDiff ==
  X : Inport
  Constant : Constant  Value=lambda1
  Constant1 : Constant  Value=alpha1
  Demux : Demux  Outputs=2
  Integrator : Integrator  InitialCondition=[0 0]
  Levant : MATLAB Function  TreatAsAtomicUnit=on
  Terminator : Terminator
  dX : Outport  VectorParamsAs1DForOutWhenUnconnected=off
  wires:
  X/1 -> Levant/2(u_ref)
  Levant/1(dX) -> Integrator/1, Demux/1
  Integrator/1 -> Levant/1(X)
  Constant/1 -> Levant/3(lambda)
  Constant1/1 -> Levant/4(alpha)
  Demux/1 -> dX/1
  Demux/2 -> Terminator/1

== system VehDynaPlayGround/Control laws/LateralController/SMC_Alcala/LevantDiff1 ==
  X : Inport
  Constant : Constant  Value=lambda1
  Constant1 : Constant  Value=alpha1
  Demux : Demux  Outputs=2
  Integrator : Integrator  InitialCondition=[0 0]
  Levant : MATLAB Function  TreatAsAtomicUnit=on
  Terminator : Terminator
  dX : Outport  VectorParamsAs1DForOutWhenUnconnected=off
  wires:
  X/1 -> Levant/2(u_ref)
  Levant/1(dX) -> Integrator/1, Demux/1
  Integrator/1 -> Levant/1(X)
  Constant/1 -> Levant/3(lambda)
  Constant1/1 -> Levant/4(alpha)
  Demux/1 -> dX/1
  Demux/2 -> Terminator/1

== matlab function VehDynaPlayGround/Tires/Tyre ModelV1/WheelsDynamic ==
  data: T_wheels input; dw_wf output; r_eff output; F_xf input; r_w parameter; r_stat parameter
% ******************* Wheel inertia dynamics *********************
%****************************************************************
% BASED ON 
% Rajesh Rajamani, Vehicle Dynamics and Control, Minneapolis, MN, Springer, 2012.
%Chapter 4.2.4
% r_eff = effective radius of the wheel
% F_xf = longitudinal tire force from the front wheels
function [dw_wf, r_eff]= fcn(T_wheels,F_xf, r_w, r_stat)

%r_w = 0.352; % radius of the tire. Pirelli Sottozero 3 P245/45WR19
%r_stat = 0.342; % static vertical deflection of the tire
alpha = acos(r_stat/r_w);
r_eff = (alpha*r_w)/alpha;

I_w = .9; % TODO define this
dw_wf = (T_wheels -(r_eff*F_xf))/I_w;

== matlab function VehDynaPlayGround/Tires/Tyre ModelV2/MagicFormula ==
  data: X input; Y output; F_zf input
%BASED ON
%Massimo Guiggiani, The Science of Vehicle Dynamics, Pisa, Italy, Springer Netherlands, 2014.
%Chapter 2.12
%The values of the MF were obtained from the graph in fig. 2.22
function Y = XTireForce(X, F_zf) 
% B stiffness factor
% C shape factor
% D peak value
% E curvature factor
% Sh horizontal shift
% Sv vertical shift

Sh = 0;% Sh horizontal shift
Sv = 0; %vertical shift

D = 3; % ym, maximum value Experimental from graph
C = 1.5;
B = 20;
E = 0;

x = X-Sh;
gamma = C*atan(B*x-E*(B*x-atan(B*x)));
y = F_zf*D*sin(gamma);
Y = (y - Sv);

== matlab function VehDynaPlayGround/Tires/Tyre ModelV2/TireSlip ==
  data: Vx input; s_xf output; w_wf input; r_eff input
%BASED ON
%Rajesh Rajamani, Vehicle Dynamics and Control, Minneapolis, MN, Springer, 2012.
%Chapter 4.1.2
function s_xf = XTireSlip(Vx,w_wf,r_eff) 

if Vx == 0
   s_xf = 0.1 * sign(w_wf);   
else
   s_xf = (r_eff*w_wf -Vx)/abs(Vx); % acceleration
end

if s_xf > 1
   %s_xf = 1; 
end

== matlab function VehDynaPlayGround/Vehicle Dynamics/LongitudinalDynamics ==
  data: F_xf input; dVx output; F_xr input; Vx input; rho parameter; g parameter; A_F parameter; C_d parameter; f parameter; m parameter; V_wind parameter; theta parameter; F_zf output; F_zr output; h_aero parameter; h_gc parameter; lf parameter; lr parameter; Nf parameter; Nr parameter
% BASED ON
% Rajesh Rajamani, Vehicle Dynamics and Control, Minneapolis, MN, Springer, 2012.
%Chapter 4.1

function [dVx,F_zf, F_zr] = LongitudinalDynamics(F_xf,F_xr,Vx, rho, g, A_F, C_d, f, m, V_wind, theta, h_aero, h_gc, lf, lr, Nf, Nr)
% m = 2238.932; % TESLA model S P85D
% g = 9.81;
% theta = 0;
% A_F = 2.341157; % Fontal area of the vehicle. TESLA model S P85D
% C_d  =0.24; %Ford Focus Aerodynamic drag coeficient. TESLA model S P85D
% rho = 1.225;  %(kg/m^3) Air density
% f = 0.01; % varies from 0.01 to 0.04
% V_wind = 0;
% Nf, Nr Number of wheels in front and rear axles

F_aero = (1/2)*rho*C_d*A_F*(Vx+V_wind)^2;

dVx = (F_xf + F_xr - F_aero - m*g*sin(theta))/m;

F_zf = (-F_aero*h_aero -m*dVx*h_gc -m*g*h_gc*sin(theta) +m*g*lr*cos(theta))/(Nf*(lr+lf));
F_zr = ( F_aero*h_aero +m*dVx*h_gc +m*g*h_gc*sin(theta) +m*g*lf*cos(theta))/(Nr*(lr+lf));

== matlab function VehDynaPlayGround/Tires/Tyre ModelV2/WheelsDynamic ==
  data: T_wheels input; dw_wf output; r_eff output; F_xf input; r_w parameter; r_stat parameter
% ******************* Wheel inertia dynamics *********************
%****************************************************************
% BASED ON 
% Rajesh Rajamani, Vehicle Dynamics and Control, Minneapolis, MN, Springer, 2012.
%Chapter 4.2.4
% r_eff = effective radius of the wheel
% F_xf = longitudinal tire force from the front wheels
function [dw_wf, r_eff]= fcn(T_wheels,F_xf, r_w, r_stat)

%r_w = 0.352; % radius of the tire. Pirelli Sottozero 3 P245/45WR19
%r_stat = 0.342; % static vertical deflection of the tire
alpha = acos(r_stat/r_w);
r_eff = (alpha*r_w)/alpha;

I_w = .9; % TODO define this
dw_wf = (T_wheels -(r_eff*F_xf))/I_w;

== matlab function VehDynaPlayGround/Vehicle Dynamics/Transmission ==
  data: T_wheels output; T_t input; w_t output; w_w input; R input
% ***************** Transmission ******************
% *************************************************
% BASED ON
% Rajesh Rajamani, Vehicle Dynamics and Control, Minneapolis, MN, Springer, 2012.
% Chapter 4.2.2
% T_wheels = wheels torque
% w_w = wheels angular speed
% R = gear ratio of transmission
%**************************************************

function [T_wheels, w_t]= fcn(T_t,w_w,R)

T_wheels = T_t/R;
w_t = w_w/R;
% itneed to be implemented "during change"

== matlab function VehDynaPlayGround/Control laws/LateralController/SMC_UrbanoPathFollowing/SMC_UrbanoPathFollowing ==
  data: U output size=1; E input; Vx input; dPsi_des input; d_d input; C_af parameter; g parameter; C_ar parameter; lf parameter; lr parameter; Iz parameter; m parameter; dd_d output
% ******************* Lateral dynamic controller *********************
%*********************************************************************
% Author: L.Arturo Torres-Romero
% Date: 22-10-2023
% This controller controlls the direction of a car, based on the path
% following controller described  in the next paper and link: 
%
%SOLEA, Razvan; NUNES, Urbano. Trajectory planning and sliding-mode control based trajectory-tracking for cybercars. 
% Integrated Computer-Aided Engineering, 2007, vol. 14, no 1, p. 33-47.
%
%https://www.researchgate.net/publication/228634486_Trajectory_planning_and_sliding-mode_control_based_trajectory-tracking_for_cybercars
%SOLEA, Razvan; NUNES, Urbano. Trajectory planning and sliding-mode control based trajectory-tracking for cybercars.
%Integrated Computer-Aided Engineering, 2007, vol. 14, no 1, p. 33-47.
%
%******************* PARAMETERS DESCRIPTIONS **********************
%******************************************************************
% m: vehicle mass
% g: gravity
% C_af : Cornering  stiffness  of  front  wheels.
% C_ar : Cornering  stiffness  of  rear  wheels.
% lf : distance fron the center of gravity to the front wheel axis.
% lr : distance fron the center of gravity to the rear wheel axis.
% Iz : this is the momentum of inertia of the vehicle respect the z axis.
%******************************************************************
%******************* INPUTS DESCRIPTIONS **************************
%******************************************************************
% E:   (column vector)[e1;de1;e2;de2] states of the state space of 
%       the system that includes the errors as follows:
%      e1  : is the lateral position error respect the road.
%      de1 : derivative of e1.
%      e2  : is the yaw angle error with respect the road. 
%      de2 : derivarive of the e2.
% Vx: Logitudinal velocity.

%******************************************************************
% ******************* OUTPUTS DESCRIPTIONS ************************
%******************************************************************
% U: control coutput in radians. Angle of the frontal wheels respect to the
%    longitudinal axis
%******************************************************************

function [U, dd_d] = SMC_Ctrl_1(E, Vx,dPsi_des, d_d, C_af, g, C_ar, lf, lr, Iz, m) % pd polos deseados
y_e = E(1);
dy_e = E(2);
psi_e = E(3);
dpsi_e = E(4);

L = lf+lr;
k = 0.5;
k0 = 0.05;
q1 = 1;
q2 = 1;
p1 = 1;
p2 = 1;
Lh = 6.5; % this lenght was obtained based in the 5 points ahead of the C.G. for refference aprx. See GetRefference block

s = dy_e + k*y_e + k0*sign(y_e)*psi_e;

if Lh == 0   % Look-ahead = 0. TODO
    ctrlVal = 0;


else   % Look-ahead <> 0|
    Q = q1;
    P = p1;
    tmp1 = (L*(cos(d_d))^2)/(Vx*Lh*cos(dpsi_e)^2);
    tmp2 = -Q*s -P*sign(s)-k*dy_e -Vx*dpsi_e*cos(psi_e) + Lh*dpsi_e^2*sin(psi_e) - k0*sign(y_e)*dpsi_e;
    dd_d = tmp1*tmp2;
    ctrlVal = real(d_d); 
end

U = real(ctrlVal);

== matlab function VehDynaPlayGround/Control laws/LateralController/AckermanCtrl ==
  data: U output size=1; E input; Vx input; C_af parameter; g parameter; C_ar parameter; lf parameter; lr parameter; Iz parameter; m parameter
% ******************* Lateral dynamic controller *********************
%*********************************************************************
% Author: L.Arturo Torres-Romero
% Date: 22-10-2020
% This controller controlls the direction of a car, based in the dynamics
% described  in the next link and using the Ackerman formulation: 
% https://www.researchgate.net/publication/340166902_LATERAL_VEHICLE_DYNAMICS_AND_CONTROLLERS_DESIGN
%******************* PARAMETERS DESCRIPTIONS **********************
%******************************************************************
% m: vehicle mass
% g: gravity
% C_af : Cornering  stiffness  of  front  wheels.
% C_ar : Cornering  stiffness  of  rear  wheels.
% lf : distance fron the center of gravity to the front wheel axis.
% lr : distance fron the center of gravity to the rear wheel axis.
% Iz : this is the momentum of inertia of the vehicle respect the z axis.
%******************************************************************
%******************* INPUTS DESCRIPTIONS **************************
%******************************************************************
% E:   (column vector)[e1;de1;e2;de2] states of the state space of 
%       the system that includes the errors as follows:
%      e1  : is the lateral position error respect the road.
%      de1 : derivative of e1.
%      e2  : is the yaw angle error with respect the road. 
%      de2 : derivarive of the e2.
% Vx: Logitudinal velocity.

%******************************************************************
% ******************* OUTPUTS DESCRIPTIONS ************************
%******************************************************************
% U: control coutput in radians. Angle of the frontal wheels respect to the
%    longitudinal axis
% isCtrl: when true means that the matrix Mc has full rank, and hence, the
%         system is controllable
%******************************************************************

function U = AckermanLateralCtrl(E, Vx, C_af, g, C_ar, lf, lr, Iz, m) % pd polos deseados
X = [0; 0; 0; 0];
X(1) = E(1);
X(2) = E(2);
X(3) = E(3);
X(4) = E(4);
%**************************************************
%******* Matrix A formulation *********************
A22 = -(2*C_af + 2*C_ar)/(m*Vx);
A23 = (2*C_af + 2*C_ar)/m;
A24 = (-2*C_af*lf + 2*C_ar*lr)/(m*Vx);
A42 = -(2*C_af*lf - 2*C_ar*lr)/(Iz*Vx);
A43 = (2*C_af*lf - 2*C_ar*lr)/Iz;
A44 = -(2*C_af*lf^2 + 2*C_ar*lr^2)/(Iz*Vx);

A = [0 1 0 0;0 A22 A23 A24;0 0 0 1;0 A42 A43 A44];
%**************************************************

%**************************************************
%******* Matrix B1 formulation ********************
B1_2 = 2*C_af/m;
B1_4 = 2*C_af*lf/Iz;

B1 = [0;B1_2;0;B1_4];
%***************************************************

%***************************************************
%******* Matrix B2 formulation *********************
B2_2 = -(2*C_af*lf - 2*C_ar*lr)/(m*Vx) - Vx;
B2_4 = -(2*C_af*lf^2 + 2*C_ar*lr^2)/(Iz*Vx);

B2 = [0;B2_2;0;B2_4];
%***************************************************


%***************************************************
%******* Matrix B3 formulation *********************
B3 = [0;g;0;0];
%***************************************************


%***************************************************
%******* Verification of controllability and output 
% calculation of the controller
%**************************************************
ctrlVal = 0;
Mc = [B1 A*B1 A^2*B1 A^3*B1];
rankVal = rank(Mc);
    if rankVal < size(A,1)
        %disp('Not completely state controllable');
        isCtrl = 0;
        ctrlVal = 0;
    else
        %disp('Completely state controllable');
        isCtrl = 1;
        % Pole placement
        Pd =[-10-3i -8+3i -15 -19]; %[-5-3i -5+3i -7 -10]
        %Pd =[-2 -2 -2 -2];

        H = (A- Pd(1)*eye(4)) * (A- Pd(2)*eye(4)) * (A- Pd(3)*eye(4)) * (A- Pd(4)*eye(4));

        %ackerman formula
        K = [0 0 0 1]*Mc^-1*H;
        ctrlVal = -K*X;  
    end


U = real(ctrlVal);

== matlab function VehDynaPlayGround/Control laws/LateralController/SMC_Alcala/LevantDiff/Levant ==
  data: dX output; X input; u_ref input; lambda input; alpha input
%*************************************************
% Author: L.Arturo Torres-Romero
% based on 
% Levant A. (1998). Robust exact differentiation via sliding mode technique. 
% Automatica, 34(3), 379-384
%*************************************************

function dX = LevantDiff(X, u_ref, lambda, alpha) 
eta_u0=X(1);    eta_u1= X(2); 

 
%Levant differenciator
 d_eta_u0=eta_u1-lambda*sqrt(abs(eta_u0-u_ref))*sign(eta_u0-u_ref);
 d_eta_u1=-alpha*sign(eta_u0-u_ref);
      
dX = [d_eta_u0;d_eta_u1];
end

== matlab function VehDynaPlayGround/Control laws/LateralController/SMC_Alcala/LevantDiff1/Levant ==
  data: dX output; X input; u_ref input; lambda input; alpha input
%*************************************************
% Author: L.Arturo Torres-Romero
% based on 
% Levant A. (1998). Robust exact differentiation via sliding mode technique. 
% Automatica, 34(3), 379-384
%*************************************************

function dX = LevantDiff(X, u_ref, lambda, alpha) 
eta_u0=X(1);    eta_u1= X(2); 

 
%Levant differenciator
 d_eta_u0=eta_u1-lambda*sqrt(abs(eta_u0-u_ref))*sign(eta_u0-u_ref);
 d_eta_u1=-alpha*sign(eta_u0-u_ref);
      
dX = [d_eta_u0;d_eta_u1];
end

== matlab function VehDynaPlayGround/Electric Actuators/SteeringActuator/BLDC_AngleCtrl/BLDC abc model ==
  data: X input; f input; v input; dX output; Tl input
function dX = fcn(X,f,v,Tl)
u = [v;Tl]; 
i_a = X(1); i_b = X(2); i_c = X(3); wm = X(4); theta = X(5);

lambda = 0.0433; %
R = 0.35;    %ohms armature resistance
L = 0.001;  %H armature inductance
M = 0.0000;  %H mutual inductance
J = 0.00018; % kgm^2 motor inertia
P = 4; % number of poles
b = 0.0034;    %Nms Hydraulic friction coefficient of motor rotor

%e = [(lamda*wm).*f;0;0];

A =[-(R/(L-M)) 0 0 -(lambda/(L-M))*f(1) 0;...
    0 -(R/(L-M)) 0 -(lambda/(L-M))*f(2) 0;...
    0 0 -(R/(L-M)) -(lambda/(L-M))*f(3) 0;...
    (lambda/J)*f(1) (lambda/J)*f(2) (lambda/J)*f(3) -b/J 0;...
    0 0 0 P/2 0];

B = diag([1/(L-M) 1/(L-M) 1/(L-M) -1/J]);
B = [B;0 0 0 0];


%dX = [0;0;0;0;0];
dX = A*X + B*u;

end
